simulink model "ascent_simulation"  (R2020a)
settings: Solver=FixedStepAuto  StartTime=0.0  StopTime=20000.0  FixedStep=dt  RelTol=1e-3
values from neighbouring files (symbols this model uses):
  balloon_drag_coeff = balloon_parameters.spec.drag_coefficient    [configure_simulation.m]    (also in linearization.m)
  box_area = 0.2 * 0.2    (= 0.04)    [configure_simulation.m]
  box_drag_coeff = 0.8    [configure_simulation.m]
  combined_dry_mass = payload_dry_mass+m_balloon    [configure_simulation.m]
  initial_altitude = 1373    [configure_simulation.m]    (also in test_kalman.m = 20000)
  parachute_area = 1.1    [configure_simulation.m]
  parachute_drag_coeff = 1.3    [configure_simulation.m]
  parachute_open_altitude = 18000    [configure_simulation.m]
libraries: simulink x1
settings Model: PacingRate=0.040000  Creator=Philip  LastModifiedBy=Philip
settings OptimizationCC: ZeroExternalMemoryAtStartup=off  ZeroInternalMemoryAtStartup=off
settings RTWCC: TargetLang=C++
settings GRTTargetCC: TargetLangStandard=C++03 (ISO)  MultiInstanceERTCode=on  CodeInterfacePackaging=C++ class

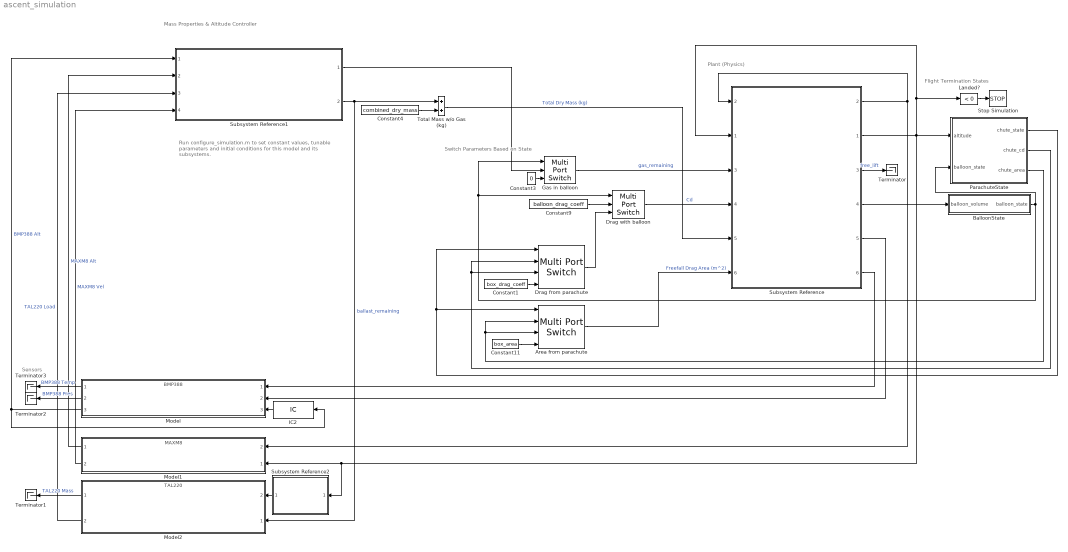
== system ascent_simulation ==
  note: Sensors
  note: Plant (Physics)
  note: Mass Properties & Altitude Controller
  note: Switch Parameters Based on State
  note: Flight Termination States
  note: Run configure_simulation.m to set constant values, tunable parameters and initial conditions for this model and its subsystems.
  Area from parachute : MultiPortSwitch  DataPortOrder=Specify indices  Inputs=4  DataPortIndices={enum_ParachuteState.FULL_OPEN, enum_ParachuteState.PART_OPEN, enum_ParachuteState.NOT_OPEN}
  BalloonState : Stateflow chart  TreatAsAtomicUnit=on
  Constant1 : Constant  Value=box_drag_coeff
  Constant11 : Constant  Value=box_area
  Constant3 : Constant  Value=0
  Constant4 : Constant  Value=combined_dry_mass
  Constant9 : Constant  Value=balloon_drag_coeff
  Drag from parachute : MultiPortSwitch  DataPortOrder=Specify indices  Inputs=4  DataPortIndices={enum_ParachuteState.FULL_OPEN, enum_ParachuteState.PART_OPEN, enum_ParachuteState.NOT_OPEN}
  Drag with balloon : MultiPortSwitch  DataPortOrder=Specify indices  Inputs=4  DataPortIndices={enum_BalloonState.INTACT, enum_BalloonState.BURST}
  Gas in balloon : MultiPortSwitch  DataPortOrder=Specify indices  Inputs=4  DataPortIndices={enum_BalloonState.INTACT, enum_BalloonState.BURST}
  IC2 : InitialCondition  Value=initial_altitude
  Landed? : simulink/Logic and Bit Operations/Compare To Zero  relop=<  OutDataTypeStr=boolean
  Model : ModelReference  ModelNameDialog=BMP388.slx  SimulationMode=Normal  ModelReferenceVersion=1.81
  Model1 : ModelReference  ModelNameDialog=MAXM8.slx  SimulationMode=Normal  ModelReferenceVersion=1.23
      settings: PortSchema="{\"entries\":[{\"content\":{\"sides\":[{\"content\":{\"connectorIds\":[\"In2\",\"In1\"]},\"type\":\"ConnectorPlacement.EquallySpacedRectSide\",\"uuid\":\"22c2536e-fdad-4c80-bedc-e4170ab07eed\"},{\"content\":{\"connectorIds\":[\"Out1\",\"Out2\"],\"side\":\"RIGHT\"},\"type\":\"ConnectorPlacement.EquallySpacedRectSide\",\"uuid\":\"eea017cd-ad84-4e64-9aef-e2df269b2e15\"},{\"content\":{\"connectorIds\":[],\"side\":\"TOP\"},\"type\":\"ConnectorPlacement.EquallySpacedRectSide\",\"uuid\":\"665077bd-e446-4439-8019-60fb4f1e3a1e\"}]},\"type\":\"ConnectorPlacement.EquallySpacedConnector\",\"uuid\":\"738747ec-ca7b-4f44-8fc9-c7c70699c607\"}],\"packageUris\":[\"http://schema.mathworks.com/mf0/Connector/19700101\"],\"version\":\"1.0\"}"
  Model2 : ModelReference  ModelNameDialog=TAL220.slx  SimulationMode=Normal  ModelReferenceVersion=1.13
      settings: PortSchema="{\"entries\":[{\"content\":{\"sides\":[{\"content\":{\"connectorIds\":[\"In2\",\"In1\"]},\"type\":\"ConnectorPlacement.EquallySpacedRectSide\",\"uuid\":\"72a1afdf-c934-47f0-b3a1-e62ce0f98852\"},{\"content\":{\"connectorIds\":[\"Out1\",\"Out2\"],\"side\":\"RIGHT\"},\"type\":\"ConnectorPlacement.EquallySpacedRectSide\",\"uuid\":\"a1e3976d-59dd-4ee9-9f8b-d4631965ab31\"},{\"content\":{\"connectorIds\":[],\"side\":\"TOP\"},\"type\":\"ConnectorPlacement.EquallySpacedRectSide\",\"uuid\":\"c6e36b0d-9981-449a-a6ab-89ba1e11611f\"}]},\"type\":\"ConnectorPlacement.EquallySpacedConnector\",\"uuid\":\"b0996c69-d360-43be-820f-b24ce198847b\"}],\"packageUris\":[\"http://schema.mathworks.com/mf0/Connector/19700101\"],\"version\":\"1.0\"}"
  ParachuteState : Stateflow chart  TreatAsAtomicUnit=on
      settings: PortSchema="{\"entries\":[{\"content\":{\"sides\":[{\"content\":{\"connectorIds\":[\"In1\",\"In2\"]},\"type\":\"ConnectorPlacement.EquallySpacedRectSide\",\"uuid\":\"9e991fac-0121-440f-aa2b-ce1063f468d8\"},{\"content\":{\"connectorIds\":[\"Out3\",\"Out2\",\"Out1\"],\"side\":\"RIGHT\"},\"type\":\"ConnectorPlacement.EquallySpacedRectSide\",\"uuid\":\"5f3b2d2b-85e8-4f00-8da4-0197870966d2\"},{\"content\":{\"connectorIds\":[],\"side\":\"TOP\"},\"type\":\"ConnectorPlacement.EquallySpacedRectSide\",\"uuid\":\"4f65fce1-3d44-4f0e-933d-bef38a38e846\"}]},\"type\":\"ConnectorPlacement.EquallySpacedConnector\",\"uuid\":\"a1c58ff8-9f3f-4e70-a348-16e72eab4418\"}],\"packageUris\":[\"http://schema.mathworks.com/mf0/Connector/19700101\"],\"version\":\"1.0\"}"
  Stop Simulation : Stop
  Subsystem Reference : Subsystem  ReferencedSubsystem=dynamics
      settings: PortSchema="{\"entries\":[{\"content\":{\"sides\":[{\"content\":{\"connectorIds\":[\"In2\",\"In1\",\"In3\",\"In4\",\"In5\",\"In6\"]},\"type\":\"ConnectorPlacement.EquallySpacedRectSide\",\"uuid\":\"164014fb-ead8-42a5-9d4d-f2559410ffa1\"},{\"content\":{\"connectorIds\":[\"Out2\",\"Out1\",\"Out3\",\"Out4\",\"Out5\",\"Out6\"],\"side\":\"RIGHT\"},\"type\":\"ConnectorPlacement.EquallySpacedRectSide\",\"uuid\":\"9bbd6586-b283-467e-9aaa-efee9e4bce66\"},{\"content\":{\"connectorIds\":[],\"side\":\"TOP\"},\"type\":\"ConnectorPlacement.EquallySpacedRectSide\",\"uuid\":\"b421fb89-32d8-4049-89c6-8e711a9b7a3e\"}]},\"type\":\"ConnectorPlacement.EquallySpacedConnector\",\"uuid\":\"ba28f21e-042f-48d8-a970-348a7e93ea1a\"}],\"packageUris\":[\"http://schema.mathworks.com/mf0/Connector/19700101\"],\"version\":\"1.0\"}"
  Subsystem Reference1 : Subsystem  ReferencedSubsystem=altitude_controller
  Subsystem Reference2 : Subsystem  ReferencedSubsystem=gravity_simple
  Terminator{,1..3} (4 alike) : Terminator
  Total Mass w/o Gas (kg) : Sum
  wires:
  Subsystem Reference/2 -> Subsystem Reference/2, Model1/2
  Total Mass w/o Gas (kg)/1 -> Subsystem Reference/5  "Total Dry Mass (kg)"
  Constant4/1 -> Total Mass w/o Gas (kg)/2
  Landed?/1 -> Stop Simulation/1
  Subsystem Reference/1 -> Subsystem Reference/1, Landed?/1, Model1/1, Subsystem Reference2/1, ParachuteState/1(altitude)
  Subsystem Reference/3 -> Terminator/1  "free_lift"
  Subsystem Reference1/2 -> Model2/1, Total Mass w/o Gas (kg)/1  "ballast_remaining"
  Subsystem Reference/4 -> BalloonState/1(balloon_volume)
  Gas in balloon/1 -> Subsystem Reference/3  "gas_remaining"
  BalloonState/1(balloon_state) -> Gas in balloon/1, Drag with balloon/1, ParachuteState/2(balloon_state)
  Constant3/1 -> Gas in balloon/3
  Subsystem Reference1/1 -> Gas in balloon/2
  Constant11/1 -> Area from parachute/4
  Constant1/1 -> Drag from parachute/4
  ParachuteState/3(chute_state) -> Drag from parachute/1, Area from parachute/1
  ParachuteState/1(chute_area) -> Area from parachute/3, Area from parachute/2
  ParachuteState/2(chute_cd) -> Drag from parachute/2, Drag from parachute/3
  Drag from parachute/1 -> Drag with balloon/3
  Drag with balloon/1 -> Subsystem Reference/4  "Cd"
  Area from parachute/1 -> Subsystem Reference/6  "Freefall Drag Area (m^2)"
  Constant9/1 -> Drag with balloon/2
  Subsystem Reference/5 -> Model/2
  Subsystem Reference/6 -> Model/1
  Model1/2 -> Subsystem Reference1/4  "MAXM8 Vel"
  Model/2 -> Terminator2/1  "BMP388 Pres"
  Model/1 -> Terminator3/1  "BMP388 Temp"
  Model/3 -> IC2/1, Subsystem Reference1/1  "BMP388 Alt"
  IC2/1 -> Model/3
  Subsystem Reference2/1 -> Model2/2
  Model2/1 -> Terminator1/1  "TAL220 Mass"
  Model1/1 -> Subsystem Reference1/2  "MAXM8 Alt"
  Model2/2 -> Subsystem Reference1/3  "TAL220 Load"

== stateflow chart ascent_simulation/BalloonState ==
  settings: stateMachineType=MOORE_MACHINE
  state Intact
    balloon_state = INTACT;
  state Burst
    balloon_state = BURST;
  (default) -> Intact
  Intact -> Burst : [balloon_volume >= burst_volume]
  data: balloon_volume input; burst_volume parameter; balloon_state output Enum: enum_BalloonState

== stateflow chart ascent_simulation/ParachuteState ==
  state Stowed
    chute_state = NOT_OPEN;
    chute_cd = 0;
    chute_area=0;
  state PartiallyDeployed
    chute_state = PART_OPEN;
    chute_cd = parachute_drag_coeff * 0.5;
    chute_area = parachute_area * 0.25;
  state FullyDeployed
    chute_state = FULL_OPEN;
    chute_cd = parachute_drag_coeff;
    chute_area = parachute_area;
  (default) -> Stowed
  Stowed -> PartiallyDeployed : [balloon_state ~= enum_BalloonState.INTACT]
  PartiallyDeployed -> FullyDeployed : [altitude < parachute_open_altitude]
  data: altitude input; parachute_open_altitude parameter; parachute_drag_coeff parameter; chute_area output; chute_cd output; chute_state output Enum: enum_ParachuteState; parachute_area parameter; balloon_state input
